simulink model "rosslerSystemLinear"  (R2019a)
settings: Solver=ode4  StartTime=0  StopTime=100  FixedStep=1e-3  RelTol=1e-3
settings Model: Creator=plazas  LastModifiedBy=plazas
settings DataIOCC: ReturnWorkspaceOutputs=off
settings OptimizationCC: DefaultParameterBehavior=Inlined
settings DebuggingCC: InitInArrayFormatMsg=none  ArithmeticOperatorsInVariantConditions=warning

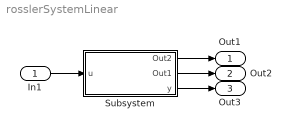
== system rosslerSystemLinear ==
  In1 : Inport
  Subsystem : Subsystem  mask{Ra=500, Rb=7500, Rc=17.5439, RCs=1, ci=[0.007026221034310 -0.035131105171551 0.035131105171551]}
      mask prompts: Ra "Resistance a"; Rb "Resistance b"; Rc "Resistance c"; RCs "Time speed (RC)"; ci "Initial Conditions"
      mask init:
      | x10 = ci(1);
      | x20 = ci(2);
      | y0 = ci(3);
      mask Display: disp("Rössler Attractor")
  Out1 : Outport
  Out2 : Outport  Port=2
  Out3 : Outport  Port=3
  wires:
  Subsystem/3("y ") -> Out3/1
  Subsystem/2(Out1) -> Out2/1
  Subsystem/1(Out2) -> Out1/1
  In1/1 -> Subsystem/1(u)

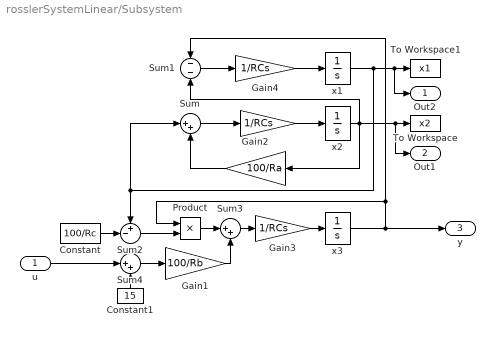
== system rosslerSystemLinear/Subsystem ==
  u : Inport
  " " : Gain  Gain=1/RCs
  Constant : Constant  Value=100/Rc
  Constant1 : Constant  Value=15
  Gain1 : Gain  Gain=100/Rb
  Gain2 : Gain  Gain=100/Ra
  Gain3 : Gain  Gain=1/RCs
  Gain4 : Gain  Gain=1/RCs
  Product : Product
  Sum : Sum  Inputs=|++
  Sum1 : Sum  Inputs=--
  Sum2 : Sum  Inputs=+-|
  Sum3 : Sum  Inputs=|++
  Sum4 : Sum  Inputs=|++
  To Workspace : ToWorkspace  VariableName=x2  SampleTime=-1
  To Workspace1 : ToWorkspace  VariableName=x1  SampleTime=-1
  x1 : Integrator  InitialCondition=x10
  x2 : Integrator  InitialCondition=x20
  "x3 " : Integrator  InitialCondition=y0
  Out2 : Outport
  Out1 : Outport  Port=2
  "y " : Outport  Port=3
  wires:
  Sum1/1 -> Gain4/1
  Gain2/1 -> Sum/2
  Sum2/1 -> Product/2
  Product/1 -> Sum3/1
  "x3 "/1 -> "y "/1, Sum1/1, Product/1
  x1/1 -> Out2/1, To Workspace1/1, Sum2/1, Sum/1
  Sum/1 -> " "/1
  Sum3/1 -> Gain3/1
  Constant/1 -> Sum2/2
  x2/1 -> Sum1/2, Out1/1, To Workspace/1, Gain2/1
  u/1 -> Sum4/1
  " "/1 -> x2/1
  Gain3/1 -> "x3 "/1
  Gain4/1 -> x1/1
  Gain1/1 -> Sum3/2
  Constant1/1 -> Sum4/2
  Sum4/1 -> Gain1/1
